simulink model "SimpleStraightLineBraking"  (R2020b)
settings: Solver=VariableStepAuto  StartTime=0.0  StopTime=10.0  MaxStep=0.01  RelTol=1e-3
undefined symbols (not defined in the file or in its folder): Input, x0
libraries: simulink x3
settings Model: Creator=Authorized User  LastModifiedBy=Authorized User

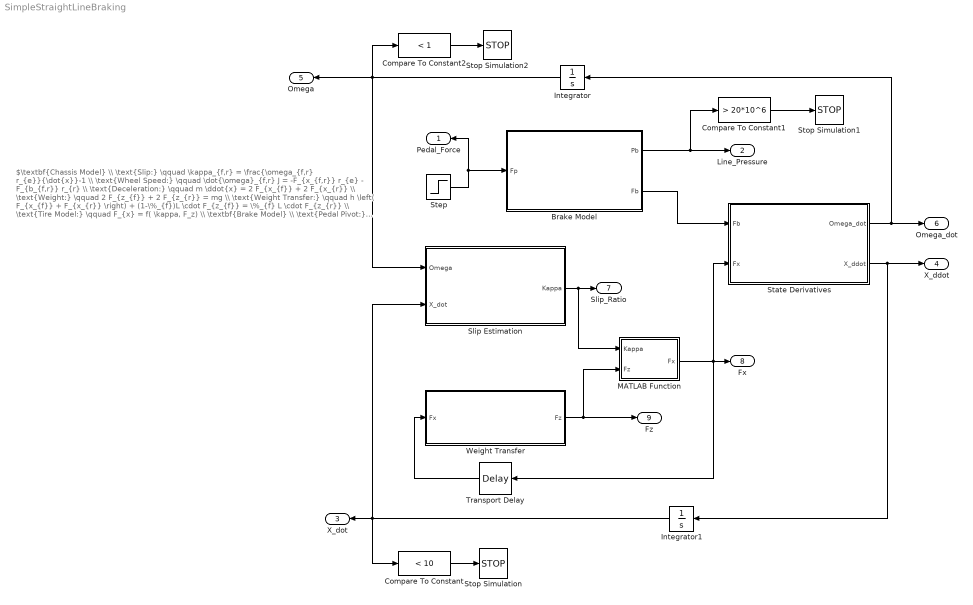
== system SimpleStraightLineBraking ==
  note: $\textbf{Chassis Model} \\ \text{Slip:} \qquad \kappa_{f,r} = \frac{\omega_{f,r} r_{e}}{\dot{x}}-1 \\ \text{Wheel Speed:} \qquad \dot{\omega}_{f,r} J = -F_{x_{f,r}} r_{e} - F_{b_{f,r}} r_{r} \\ \text{Deceleration:} \qquad m \ddot{x} = 2 F_{x_{f}} + 2 F_{x_{r}} \\ \text{Weight:} \qquad 2 F_{z_{f}} + 2 F_{z_{r}} = mg \\ \text{Weight Transfer:} \qquad h \left( F_{x_{f}} + F_{x_{r}} \right) + (1-\%_{f})L \cdot F_{z_{f}} = \%_{f} L \cdot F_{z_{r}} \\ \text{Tire Model:} \qquad F_{x} = f( \kappa, F_z) \\ \textbf{Brake Model} \\ \text{Pedal Pivot:} \qquad F_{p} \cdot \eta(\theta_{p}) = \left( F_{c_{f}} + F_{c_{r}} \right) \\ \text{Balance Bar:} \qquad F_{c_{f}} \cdot (1 - \%_{bb}) = F_{c_{r}} \cdot \%_{bb}\\ \text{Cylinder, Line, & Pad:} \qquad 2F_{b_{f,r}} = F_{c_{f,r}} \frac{A_{p} \mu_{p}}{\frac{\pi}{4} D_{b_{f,r}}^{2}} \\$
  Brake Model : MATLAB Function  TreatAsAtomicUnit=on
  Compare To Constant : simulink/Logic and Bit Operations/Compare To Constant  relop=<  const=10  OutDataTypeStr=boolean
  Compare To Constant1 : simulink/Logic and Bit Operations/Compare To Constant  relop=>  const=20*10^6  OutDataTypeStr=boolean
  Compare To Constant2 : simulink/Logic and Bit Operations/Compare To Constant  relop=<  const=1  OutDataTypeStr=boolean
  Integrator : Integrator  InitialCondition=x0(2:3)
  Integrator1 : Integrator  InitialCondition=x0(1)
  MATLAB Function : MATLAB Function  TreatAsAtomicUnit=on
  Slip Estimation : MATLAB Function  TreatAsAtomicUnit=on
  State Derivatives : MATLAB Function  TreatAsAtomicUnit=on
  Step : Step  Time=0.1  After=Input.Fp  SampleTime=0
  Stop Simulation : Stop
  Stop Simulation1 : Stop
  Stop Simulation2 : Stop
  Transport Delay : TransportDelay  DelayTime=0.005
  Weight Transfer : MATLAB Function  TreatAsAtomicUnit=on
  Pedal_Force : Outport
  Line_Pressure : Outport  Port=2
  X_dot : Outport  Port=3
  X_ddot : Outport  Port=4
  Omega : Outport  Port=5
  Omega_dot : Outport  Port=6
  Slip_Ratio : Outport  Port=7
  Fx : Outport  Port=8
  Fz : Outport  Port=9
  wires:
  Integrator/1 -> Compare To Constant2/1, Slip Estimation/1(Omega), Omega/1
  State Derivatives/2(X_ddot) -> Integrator1/1, X_ddot/1
  Integrator1/1 -> Compare To Constant/1, X_dot/1, Slip Estimation/2(X_dot)
  Step/1 -> Pedal_Force/1, Brake Model/1(Fp)
  Weight Transfer/1(Fz) -> MATLAB Function/2(Fz), Fz/1
  Brake Model/1(Pb) -> Compare To Constant1/1, Line_Pressure/1
  Brake Model/2(Fb) -> State Derivatives/1(Fb)
  State Derivatives/1(Omega_dot) -> Omega_dot/1, Integrator/1
  MATLAB Function/1(Fx) -> Transport Delay/1, Fx/1, State Derivatives/2(Fx)
  Slip Estimation/1(Kappa) -> MATLAB Function/1(Kappa), Slip_Ratio/1
  Transport Delay/1 -> Weight Transfer/1(Fx)
  Compare To Constant/1 -> Stop Simulation/1
  Compare To Constant1/1 -> Stop Simulation1/1
  Compare To Constant2/1 -> Stop Simulation2/1

== matlab function SimpleStraightLineBraking/Weight Transfer ==
  data: Fx input; Fz output; Parameter parameter
function Fz = WeightTransfer(Fx, Parameter)

Fz = [2 2; -(1-Parameter.Mass.pf) Parameter.Mass.pf] \ ...
    [Parameter.Mass.m .* 9.81; Parameter.Mass.h ./ Parameter.Susp.L .* sum(Fx) ];

== matlab function SimpleStraightLineBraking/Brake Model ==
  data: Pb output; Fb output; Fp input; Parameter parameter
function [Pb, Fb] = BrakeModel(Fp, Parameter)

%% Evaluate Brake Forces
Fc = [1, 1; (1-Parameter.Pedal.pbb), -Parameter.Pedal.pbb] \ ...
    [Parameter.Pedal.eta .* Fp, 0]';

Pb = Fc ./ ( pi/4 .* Parameter.Brake.Db.^2 );
Fb = Pb/2 .* Parameter.Brake.Ap .* Parameter.Brake.mu;

== matlab function SimpleStraightLineBraking/Slip Estimation ==
  data: Omega input; X_dot input; Kappa output; Parameter parameter
function Kappa  = SlipEstimation(Omega, X_dot, Parameter)

%% Slip Estimation
Kappa = Omega .* Parameter.Re ./ X_dot - 1;

== matlab function SimpleStraightLineBraking/State Derivatives ==
  data: Fb input; Omega_dot output; Fx input; Parameter parameter; X_ddot output
function [Omega_dot, X_ddot] = BrakeModel(Fb, Fx, Parameter)

%% Evaluate Accelerations
Omega_dot = (-Fx .* Parameter.Re - Fb .* Parameter.Brake.Rr ) / ...
    Parameter.Wheel.J;

X_ddot = 2 .* sum( Fx ) / Parameter.Mass.m;

== matlab function SimpleStraightLineBraking/MATLAB Function ==
  data: Kappa input; Fx output size=[2]; Fz input; Parameter parameter
function Fx = TireModel(Kappa, Fz, Parameter)
Pi = 80;
Inc = 0;

dFz = (Fz - Parameter.Pacejka.Fzo) ./ Parameter.Pacejka.Fzo;
dPi = (Pi - Parameter.Pacejka.Pio) ./ Parameter.Pacejka.Pio;

Cx = Parameter.Pacejka.p.C.x(1) .* Parameter.Pacejka.L.C.x;

Dx = (Parameter.Pacejka.p.D.x(1) + Parameter.Pacejka.p.D.x(2).*dFz) .* ...
     (1 + Parameter.Pacejka.p.P.x(3).*dPi + Parameter.Pacejka.p.P.x(4).*dPi.^2) .* ...
     (1 - Parameter.Pacejka.p.D.x(3).*Inc.^2).*Fz .* Parameter.Pacejka.L.mu.x;

Ex = ( Parameter.Pacejka.p.E.x(1) + Parameter.Pacejka.p.E.x(2).*dFz ...
    + Parameter.Pacejka.p.E.x(3).*dFz.^2 ) .* ( 1 - Parameter.Pacejka.p.E.x(4).*sign(Kappa) ) .* ...
    Parameter.Pacejka.L.E.x;

Kxk = Fz.*(Parameter.Pacejka.p.K.x(1) + Parameter.Pacejka.p.K.x(2).*dFz ) .* ...
    exp( Parameter.Pacejka.p.K.x(3) .* dFz ) .* ...
    (1 + Parameter.Pacejka.p.P.x(1).*dPi + Parameter.Pacejka.p.P.x(2).*dPi.^2) .* ...
    Parameter.Pacejka.L.K.x.k;

Bx = Kxk ./ ( Cx.*Dx );

Vx = Fz.*(Parameter.Pacejka.p.V.x(1) + Parameter.Pacejka.p.V.x(2).*dFz ) .* ...
    Parameter.Pacejka.L.V.x;

Hx = (Parameter.Pacejka.p.H.x(1) + Parameter.Pacejka.p.H.x(2).*dFz) .* ...
    Parameter.Pacejka.L.H.x;

Fx = Dx .* sin( Cx .* atan( (1-Ex) .* Bx.*(Kappa + Hx) + ...
    Ex.*atan( Bx.*(Kappa + Hx) ) ) ) + Vx;
